simulink model "Sistema_Desarrollado"  (R2015b)
settings: Solver=FixedStepDiscrete  StartTime=0.0  StopTime=1000  RelTol=1e-3
libraries: libreria_temas_3y4 x2
settings Model: Creator=AJA  LastModifiedBy=Shagai
settings DataIOCC: SaveFormat=Array  SignalLoggingSaveFormat=ModelDataLogs
settings OptimizationCC: ExpressionDepthLimit=2147483647  InitFltsAndDblsToZero=on
settings DebuggingCC: UnderspecifiedInitializationDetection=Classic  MergeDetectMultiDrivingBlocksExec=none  SolverPrmCheckMsg=warning  FcnCallInpInsideContextMsg=UseLocalSettings  StateNameClashWarn=warning
settings HardwareCC: ProdBitPerPointer=32  ProdLargestAtomicFloat=None  ProdIntDivRoundTo=Undefined  ProdEndianess=Unspecified  ProdWordSize=32  ProdHWDeviceType=32-bit Generic  TargetHWDeviceType=32-bit Generic
settings GRTTargetCC: TargetFcnLib=ansi_tfl_tmw.mat  GeneratePreprocessorConditionals=Disable all  CombineOutputUpdateFcns=off  GRTInterface=on
settings ConfigComp: CovModelRefEnable=Off

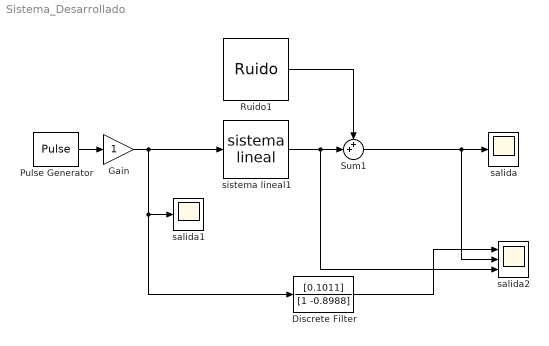
== system Sistema_Desarrollado ==
  Discrete Filter : DiscreteFilter  Numerator=[0.1011]  Denominator=[1 -0.8988]
  Gain : Gain
  Pulse Generator : DiscretePulseGenerator  Amplitude=80  Period=200  PulseWidth=100  SampleTime=0.1
  Ruido1 : libreria_temas_3y4/Ruido
  Sum1 : Sum  Inputs=++|
  salida : Scope
  salida1 : Scope
  salida2 : Scope  NumInputPorts=3
  sistema lineal1 : libreria_temas_3y4/sistema lineal
  wires:
  Pulse Generator/1 -> Gain/1
  sistema lineal1/1 -> salida2/3, Sum1/2
  Gain/1 -> Discrete Filter/1, salida1/1, sistema lineal1/1
  Ruido1/1 -> Sum1/1
  Sum1/1 -> salida2/2, salida/1
  Discrete Filter/1 -> salida2/1
